simulink model "chorus"  (R2024a)
settings: Solver=VariableStepAuto  StartTime=0.0  StopTime=20  RelTol=1e-3
libraries: dspsnks4 x1, hdlsllib x1, dspvision x1
settings Model: Creator=fermata  LastModifiedBy=fermata
settings OptimizationCC: BlockReduction=off  ConditionallyExecuteInputs=off

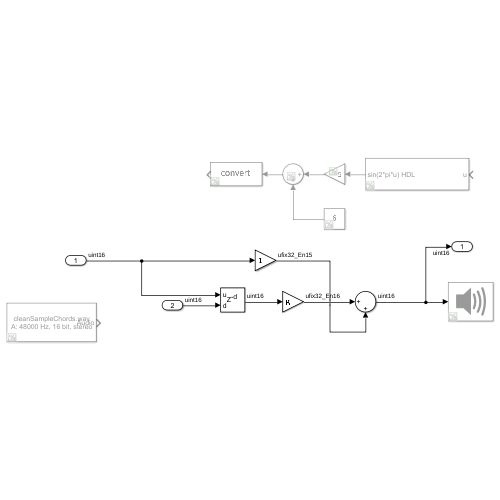
[thumbnail: Simulink's stored preview of the top-level diagram]
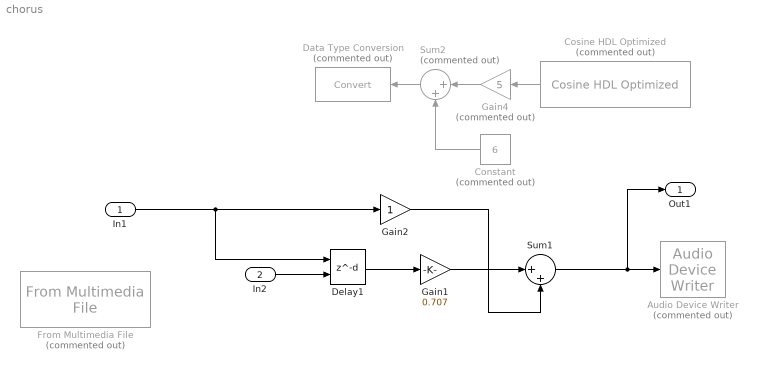
== system chorus ==
  In1 : Inport  OutDataTypeStr=uint16
  In2 : Inport  Port=2  OutDataTypeStr=uint16
  Audio Device Writer : dspsnks4/Audio Device Writer  Commented=on  Driver=ALSA  Device=Default  InheritSampleRate=on  SampleRate=44100  BitDepth=16-bit integer  BufferSize=4096  NumBuffers=10  DefaultOutputChannelMapping=on  OutputChannelMapping=1:2  OutputNumUnderrunSamples=off  DriverIdx=8  DeviceWarnFlag=''
  Constant : Constant  Commented=on  Value=6  OutDataTypeStr=int16
  Cosine HDL Optimized : hdlsllib/Lookup Tables/Cosine HDL Optimized  Commented=on  OutputFormula=sin(2*pi*u)  NumDataPoints=65536  TableDataTypeStr=fixdt(0,16,15)  SimulateLUTROMDelay=off
  Data Type Conversion : DataTypeConversion  Commented=on  RndMeth=Round  SaturateOnIntegerOverflow=off
  Delay1 : Delay  DelayLengthSource=Input port  DelayLength=1  DelayLengthUpperLimit=1024  InitialCondition=0
      settings: InputPortMap=u0,p1
  From Multimedia File : dspvision/From Multimedia File  Commented=on  inputFilename=/home/fermata/Development/FPGA/patatodsp/doc/ADSD/Code/examples/simulink-common/cleanSampleChords.wav  readRange=[1 Inf]  loop=on  numPlays=inf  outputStreams=Audio only  videoDataType=single  audioDataType=int16  inheritSampleTime=on  userDefinedSampleTime=1/30  noAudioOutput=off  isIntensityVideo=off  fourcc=RGB  colorVideoFormat=Separate color signals  outputEOF=off  dataOrg=Column-major  audioFrameSize=1024  computeAudioFrameSize=off  outSamplingMode=Sample based
      settings: LibrarySourceBlock=audiosources/From Multimedia File
  Gain1 : Gain  Gain=0.707
  Gain2 : Gain
  Gain4 : Gain  Commented=on  Gain=5  OutDataTypeStr=int16  RndMeth=Round  SaturateOnIntegerOverflow=on
  Sum1 : Sum  Inputs=|++  OutDataTypeStr=uint16  RndMeth=Round  SaturateOnIntegerOverflow=on
  Sum2 : Sum  Commented=on  Inputs=|++
  Out1 : Outport  OutDataTypeStr=uint16
  wires:
  Delay1/1 -> Gain1/1
  Gain1/1 -> Sum1/1
  Gain2/1 -> Sum1/2
  Sum1/1 -> Out1/1, Audio Device Writer/1
  Gain4/1 -> Sum2/1
  Cosine HDL Optimized/1 -> Gain4/1
  Sum2/1 -> Data Type Conversion/1
  Constant/1 -> Sum2/2
  In1/1 -> Gain2/1, Delay1/1
  In2/1 -> Delay1/2
